simulink model "TDsimulation"  (Simulink 8.3)
settings: Solver=ode4  StartTime=0.0  StopTime=Tsim  FixedStep=Ts  RelTol=1e-3
InitFcn:
  | GlobalParam;
values from neighbouring files (symbols this model uses):
  APFon = 0.02    [GlobalParam.m]
  Cdc = 680e-6    (= 0.00068)    [GlobalParam.m]
  fe = 50    [GlobalParam.m]
  Ideal = 0    [GlobalParam.m]
  Lf = 0.002996    [GlobalParam.m]
  LL = 0.055462    [GlobalParam.m]
  Rf = 0.09    [GlobalParam.m]
  RL = 23.232    [GlobalParam.m]
  tetaa = 0    [GlobalParam.m]
  tetab = -120    [GlobalParam.m]
  tetac = 120    [GlobalParam.m]
  Tm = 1/fm    (= 0.0001)    [GlobalParam.m]
  Ts = 1e-6    (= 1e-06)    [GlobalParam.m]
  Vdc = 114    [GlobalParam.m]
  Vs = 310.2    [GlobalParam.m]
libraries: powerlib x115, powerlib_extras x3
(part 1 of 2)
settings Model: Creator=User  LastModifiedBy=Leocompa
settings OptimizationCC: ExpressionDepthLimit=2147483647
settings DebuggingCC: FcnCallInpInsideContextMsg=EnableAllAsWarning
settings GRTTargetCC: CombineOutputUpdateFcns=on  GRTInterface=off

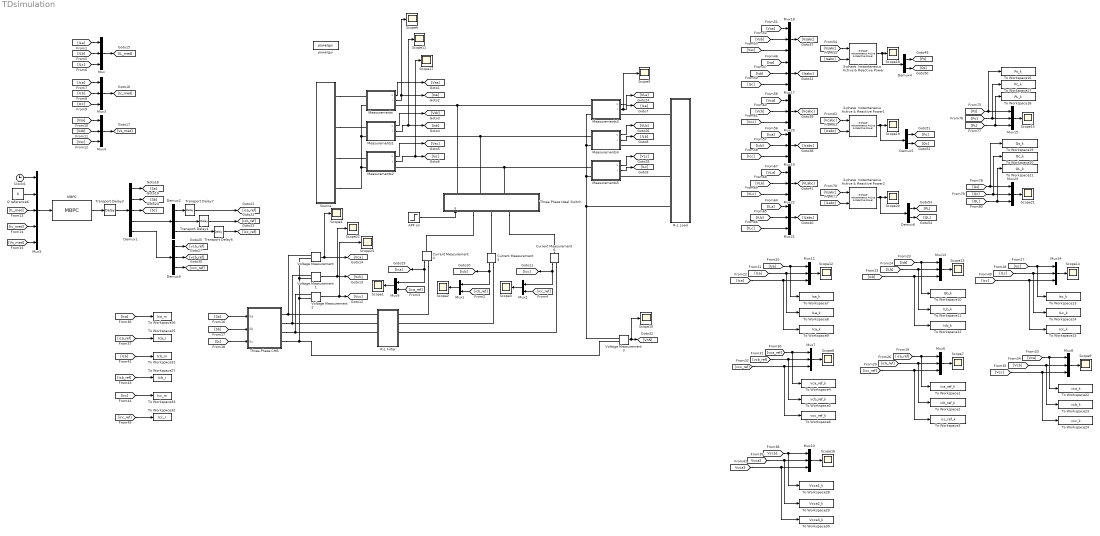
== system TDsimulation ==
  3-phase  Instantaneous  Active & Reactive Power : powerlib_extras/Measurements/3-phase  Instantaneous  Active & Reactive Power
  3-phase  Instantaneous  Active & Reactive Power1 : powerlib_extras/Measurements/3-phase  Instantaneous  Active & Reactive Power
  3-phase  Instantaneous  Active & Reactive Power2 : powerlib_extras/Measurements/3-phase  Instantaneous  Active & Reactive Power
  APF on : Step  Time=APFon  SampleTime=0
  Clock6 : Clock
  Current Measurement4 : powerlib/Measurements/Current Measurement  PhasorSimulation=off  OutputType=Complex  PSBequivalent=0
  Current Measurement5 : powerlib/Measurements/Current Measurement  PhasorSimulation=off  OutputType=Complex  PSBequivalent=0
  Current Measurement6 : powerlib/Measurements/Current Measurement  PhasorSimulation=off  OutputType=Complex  PSBequivalent=0
  Demux1 : Demux  Outputs=5
  Demux2 : Demux  Outputs=3
  Demux4 : Demux  Outputs=2
  Demux5 : Demux  Outputs=2
  Demux6 : Demux  Outputs=2
  Demux9 : Demux  Outputs=3
  MBPC : MATLABFcn  MATLABFcn=MBPC  OutputDimensions=24
  Measurements : Subsystem
  Measurements1 : Subsystem
  Measurements2 : Subsystem
  Measurements3 : Subsystem
  Measurements4 : Subsystem
  Measurements5 : Subsystem
  Mux{,3..4,6..8,10,12..15,17..23} (18 alike) : Mux  Inputs=3
  Mux1 : Mux  Inputs=2
  Mux2 : Mux  Inputs=2
  Mux5 : Mux  Inputs=5
  Mux9 : Mux  Inputs=2
  Q reference6 : Constant  Value=0
  R-L Filter : Subsystem
  R-L Load : Subsystem
  Scope{1..23} (23 alike) : Scope
      Scope1 settings: YMin=-15  YMax=65  SaveName=Vo
      Scope10 settings: YMin=-2500  YMax=37500  SaveName=vNn
      Scope11 settings: YMin=-10.7  YMax=-9.4  SaveName=isb
      Scope12 settings: YMin=-11  YMax=11  SaveName=Vo11
      Scope13 settings: YMin=-11  YMax=11  SaveName=Vo12
      Scope14 settings: YMin=25  YMax=575  SaveName=Vo13
      Scope15 settings: YMin=-750  YMax=4250  SaveName=Vo14
      Scope16 settings: TimeRange=0.1  YMin=27.5  YMax=75  SaveName=Vo15
      Scope17 settings: YMin=-10.7  YMax=-9.4  SaveName=isc
      Scope18 settings: YMin=-1500  YMax=5500  SaveName=Vo17
      Scope19 settings: YMin=-1500  YMax=5500  SaveName=Vo18
      Scope2 settings: YMin=-2.5  YMax=6.5  SaveName=Vo1
      Scope20 settings: YMin=-1500  YMax=5500  SaveName=Vo19
      Scope21 settings: TimeRange=0.1  YMin=-400  YMax=4000  SaveName=Vo20
      Scope22 settings: YMin=-2500  YMax=37500  SaveName=vcb
      Scope23 settings: YMin=-2500  YMax=37500  SaveName=vcc
      Scope3 settings: YMin=-2.5  YMax=6.5  SaveName=Vo2
      Scope4 settings: YMin=-2500  YMax=37500  SaveName=vca
      Scope5 settings: YMin=-2500  YMax=37500  SaveName=iLa
      Scope6 settings: YMin=-10.7  YMax=-9.4  SaveName=isa
      Scope7 settings: YMin=25  YMax=575  SaveName=Vo6
      Scope8 settings: YMin=25  YMax=575  SaveName=Vo7
      Scope9 settings: YMin=25  YMax=575  SaveName=Vo8
  Source : Subsystem
  Three-Phase CHB : Subsystem
  Three-Phase Ideal Switch : Subsystem
  To Workspace1 : ToWorkspace  VariableName=ica_ref_k  SaveFormat=Timeseries  SampleTime=-1
  To Workspace10 : ToWorkspace  VariableName=Isb_k  SaveFormat=Timeseries  SampleTime=-1
  To Workspace11 : ToWorkspace  VariableName=ILb_k  SaveFormat=Timeseries  SampleTime=-1
  To Workspace12 : ToWorkspace  VariableName=Icb_k  SaveFormat=Timeseries  SampleTime=-1
  To Workspace13 : ToWorkspace  VariableName=Isc_k  SaveFormat=Timeseries  SampleTime=-1
  To Workspace14 : ToWorkspace  VariableName=ILc_k  SaveFormat=Timeseries  SampleTime=-1
  To Workspace15 : ToWorkspace  VariableName=Icc_k  SaveFormat=Timeseries  SampleTime=-1
  To Workspace16 : ToWorkspace  VariableName=Ps_k  SaveFormat=Timeseries  SampleTime=-1
  To Workspace17 : ToWorkspace  VariableName=Pc_k  SaveFormat=Timeseries  SampleTime=-1
  To Workspace18 : ToWorkspace  VariableName=PL_k  SaveFormat=Timeseries  SampleTime=-1
  To Workspace19 : ToWorkspace  VariableName=Qs_k  SaveFormat=Timeseries  SampleTime=-1
  To Workspace2 : ToWorkspace  VariableName=icb_ref_k  SaveFormat=Timeseries  SampleTime=-1
  To Workspace20 : ToWorkspace  VariableName=Qc_k  SaveFormat=Timeseries  SampleTime=-1
  To Workspace21 : ToWorkspace  VariableName=QL_k  SaveFormat=Timeseries  SampleTime=-1
  To Workspace22 : ToWorkspace  VariableName=vca_k  SaveFormat=Timeseries  SampleTime=-1
  To Workspace23 : ToWorkspace  VariableName=vcb_k  SaveFormat=Timeseries  SampleTime=-1
  To Workspace24 : ToWorkspace  VariableName=vcc_k  SaveFormat=Timeseries  SampleTime=-1
  To Workspace25 : ToWorkspace  VariableName=Ica_r  SampleTime=-1
  To Workspace26 : ToWorkspace  VariableName=Ica_m  SampleTime=-1
  To Workspace27 : ToWorkspace  VariableName=Icb_r  SampleTime=-1
  To Workspace28 : ToWorkspace  VariableName=Vcca1_k  SaveFormat=Timeseries  SampleTime=-1
  To Workspace29 : ToWorkspace  VariableName=Vcca2_k  SaveFormat=Timeseries  SampleTime=-1
  To Workspace3 : ToWorkspace  VariableName=icc_ref_k  SaveFormat=Timeseries  SampleTime=-1
  To Workspace30 : ToWorkspace  VariableName=Vcca3_k  SaveFormat=Timeseries  SampleTime=-1
  To Workspace31 : ToWorkspace  VariableName=Icb_m  SampleTime=-1
  To Workspace32 : ToWorkspace  VariableName=Icc_r  SampleTime=-1
  To Workspace33 : ToWorkspace  VariableName=Icc_m  SampleTime=-1
  To Workspace4 : ToWorkspace  VariableName=vca_ref_k  SaveFormat=Timeseries  SampleTime=-1
  To Workspace5 : ToWorkspace  VariableName=vcb_ref_k  SaveFormat=Timeseries  SampleTime=-1
  To Workspace6 : ToWorkspace  VariableName=vcc_ref_k  SaveFormat=Timeseries  SampleTime=-1
  To Workspace7 : ToWorkspace  VariableName=Isa_k  SaveFormat=Timeseries  SampleTime=-1
  To Workspace8 : ToWorkspace  VariableName=ILa_k  SaveFormat=Timeseries  SampleTime=-1
  To Workspace9 : ToWorkspace  VariableName=Ica_k  SaveFormat=Timeseries  SampleTime=-1
  Transport Delay{3..4,6..7} (4 alike) : TransportDelay  DelayTime=Tm
  Voltage Measurement{,1..3} (4 alike) : powerlib/Measurements/Voltage Measurement  PhasorSimulation=off  OutputType=Complex  PSBequivalent=0
  powergui : powerlib/powergui  SimulationMode=Discrete  SolverType=Backward Euler  SampleTime=Ts  frequency=60  SPID=off  DisableSnubberDevices=off  DisableRonSwitches=off  DisableVfSwitches=off  SwTol=0  Interpol=off  DisplayEquations=off  Ts=0  methode=off  frequencyindice=0  Pbase=100e6  ErrMax=1e-4  Iterations=50  UnitsV=kV  UnitsW=MW  FunctionMessages=off  echomessages=off  HookPort=off  EnableUseOfTLC=off  x0status=blocks  RestoreLinks=warning  ResistiveCurrentMeasurement=off  Frange=[0:2:500]  Ylog=off  Xlog=on  ShowGrid=off  save=off  variable=ZData  structure=vcc  ZoomFFT=off  StartTime=0.03  cycles=2  DisplayStyle=1  fundamental=50  FreqAxis=off  MaxFrequency=60000  frequencyindicesteady=1  RmsSteady=1  display=off
  wires:
  Measurements/2(i) -> Scope6/1, [Isa]
  Measurements/1(v) -> [Vsa]
  Measurements1/1(v) -> [Vsb]
  Measurements2/1(v) -> [Vsc]
  Current Measurement4/1 -> Mux9/1, [Ica]
  Mux9/1 -> Scope1/1
  [ica_ref] -> Mux9/2
  Current Measurement5/1 -> Mux1/1, [Icb]
  Mux1/1 -> Scope2/1
  [icb_ref] -> Mux1/2
  Current Measurement6/1 -> Mux2/1, [Icc]
  Mux2/1 -> Scope3/1
  [icc_ref] -> Mux2/2
  Voltage Measurement/1 -> [Vca], Scope4/1
  Voltage Measurement2/1 -> Scope23/1, [Vcc]
  APF on/1 -> Three-Phase Ideal Switch/1(g)
  [ILa] -> Mux/1
  [ILb] -> Mux/2
  [ILc] -> Mux/3
  [Ica] -> Mux3/1
  [Icb] -> Mux3/2
  [Icc] -> Mux3/3
  [Vsa] -> Mux4/1
  [Vsb] -> Mux4/2
  [Vsc] -> Mux4/3
  Mux/1 -> [IL_med]
  Mux3/1 -> [Ic_med]
  Mux4/1 -> [Vs_med]
  [Sa] -> Three-Phase CHB/1(Sa)
  [Sb] -> Three-Phase CHB/2(Sb)
  [Sc] -> Three-Phase CHB/3(Sc)
  [Icb] -> Mux13/3, To Workspace12/1
  Mux12/1 -> Scope12/1
  Mux13/1 -> Scope13/1
  [Isc] -> Mux14/1, To Workspace13/1
  [Ica] -> Mux12/3, To Workspace9/1
  [ILc] -> Mux14/2, To Workspace14/1
  [Isa] -> Mux12/1, To Workspace7/1
  [ILb] -> Mux13/2, To Workspace11/1
  Mux14/1 -> Scope14/1
  [Icc] -> Mux14/3, To Workspace15/1
  [ILa] -> Mux12/2, To Workspace8/1
  [Isb] -> Mux13/1, To Workspace10/1
  [ica_ref] -> Mux6/1, To Workspace1/1
  [icb_ref] -> Mux6/2, To Workspace2/1
  Mux6/1 -> Scope7/1
  [icc_ref] -> Mux6/3, To Workspace3/1
  Demux6/1 -> [PL]
  Demux5/1 -> [Pc]
  Demux5/2 -> [Qc]
  [Isabc] -> 3-phase  Instantaneous  Active & Reactive Power/2
  [Vsb] -> Mux18/2
  [Ica] -> Mux19/1
  Mux17/1 -> [Isabc]
  Demux6/2 -> [QL]
  Demux4/1 -> [Ps]
  Demux4/2 -> [Qs]
  [ILc] -> Mux21/3
  Mux19/1 -> [Icabc]
  [PL] -> Mux15/3, To Workspace18/1
  [Pc] -> Mux15/2, To Workspace17/1
  [Icc] -> Mux19/3
  [Qc] -> Mux23/2, To Workspace20/1
  Mux21/1 -> [ILabc]
  [Qs] -> Mux23/1, To Workspace19/1
  [Isb] -> Mux17/2
  Mux18/1 -> [Vsabc]
  [Isc] -> Mux17/3
  [Vsabc] -> 3-phase  Instantaneous  Active & Reactive Power/1
  [ILa] -> Mux21/1
  Mux20/1 -> [Vcabc]
  [ILb] -> Mux21/2
  3-phase  Instantaneous  Active & Reactive Power2/1 -> Scope20/1, Demux6/1
  3-phase  Instantaneous  Active & Reactive Power1/1 -> Scope19/1, Demux5/1
  Mux22/1 -> [VLabc]
  [Vsa] -> Mux18/1
  [Vsabc] -> 3-phase  Instantaneous  Active & Reactive Power2/1
  Mux15/1 -> Scope15/1
  [ILabc] -> 3-phase  Instantaneous  Active & Reactive Power2/2
  [Vcc] -> Mux20/3
  Mux23/1 -> Scope21/1
  [Icabc] -> 3-phase  Instantaneous  Active & Reactive Power1/2
  [Icb] -> Mux19/2
  [VLc] -> Mux22/3
  [Isa] -> Mux17/1
  [Vcb] -> Mux20/2
  [Vsc] -> Mux18/3
  [Vca] -> Mux20/1
  [VLa] -> Mux22/1
  [Ps] -> Mux15/1, To Workspace16/1
  [VLb] -> Mux22/2
  3-phase  Instantaneous  Active & Reactive Power/1 -> Scope18/1, Demux4/1
  [QL] -> Mux23/3, To Workspace21/1
  [Vcabc] -> 3-phase  Instantaneous  Active & Reactive Power1/1
  Measurements3/2(i) -> Scope5/1, [ILa]
  Measurements3/1(v) -> [VLa]
  Measurements4/2(i) -> [ILb]
  Measurements4/1(v) -> [VLb]
  Measurements5/2(i) -> [ILc]
  Measurements5/1(v) -> [VLc]
  [vca_ref] -> Mux7/1, To Workspace4/1
  [vcb_ref] -> Mux7/2, To Workspace5/1
  Mux7/1 -> Scope8/1
  [vcc_ref] -> Mux7/3, To Workspace6/1
  [Vca] -> Mux8/1, To Workspace22/1
  [Vcb] -> Mux8/2, To Workspace23/1
  Mux8/1 -> Scope9/1
  [Vcc] -> Mux8/3, To Workspace24/1
  Voltage Measurement3/1 -> Scope10/1, [VnN]
  [Ica] -> To Workspace26/1
  [ica_ref] -> To Workspace25/1
  Mux10/1 -> Scope16/1
  [Vcca1] -> Mux10/1, To Workspace28/1
  [Vcca2] -> Mux10/2, To Workspace29/1
  [Vcca3] -> Mux10/3, To Workspace30/1
  Measurements1/2(i) -> Scope11/1, [Isb]
  Measurements2/2(i) -> [Isc], Scope17/1
  [Icb] -> To Workspace31/1
  [icb_ref] -> To Workspace27/1
  [Icc] -> To Workspace33/1
  [icc_ref] -> To Workspace32/1
  Voltage Measurement1/1 -> [Vcb], Scope22/1
  Mux5/1 -> MBPC/1
  [IL_med] -> Mux5/3
  [Ic_med] -> Mux5/4
  [Vs_med] -> Mux5/5
  Q reference6/1 -> Mux5/2
  Clock6/1 -> Mux5/1
  Demux9/3 -> [vcc_ref]
  Demux9/2 -> [vcb_ref]
  Demux9/1 -> [vca_ref]
  Demux1/1 -> [Sa]
  Demux1/2 -> [Sb]
  Demux1/3 -> [Sc]
  Demux1/4 -> Demux2/1
  Demux1/5 -> Demux9/1
  Transport Delay3/1 -> Demux1/1
  MBPC/1 -> Transport Delay3/1
  Demux2/1 -> Transport Delay7/1
  Demux2/2 -> Transport Delay4/1
  Demux2/3 -> Transport Delay6/1
  Transport Delay6/1 -> [icc_ref]
  Transport Delay7/1 -> [ica_ref]
  Transport Delay4/1 -> [icb_ref]
  connections:
  Source/RConn3 -- Measurements2/LConn1
  Source/RConn2 -- Measurements1/LConn1
  Source/RConn1 -- Measurements/LConn1
  Measurements/LConn2 -- Source/RConn4 -- Measurements2/LConn2 -- Measurements1/LConn2
  Three-Phase Ideal Switch/RConn1 -- Measurements3/LConn1 -- Measurements/RConn1
  Three-Phase Ideal Switch/RConn2 -- Measurements4/LConn1 -- Measurements1/RConn1
  Three-Phase Ideal Switch/RConn3 -- Measurements5/LConn1 -- Measurements2/RConn1
  Current Measurement4/RConn1 -- R-L Filter/RConn1
  Current Measurement5/RConn1 -- R-L Filter/RConn2
  Current Measurement6/RConn1 -- R-L Filter/RConn3
  Three-Phase Ideal Switch/LConn2 -- Current Measurement5/LConn1
  Three-Phase Ideal Switch/LConn3 -- Current Measurement6/LConn1
  Three-Phase Ideal Switch/LConn1 -- Current Measurement4/LConn1
  Voltage Measurement/LConn2 -- Voltage Measurement1/LConn2 -- Voltage Measurement2/LConn2 -- Voltage Measurement3/LConn2 -- Three-Phase CHB/RConn4
  Three-Phase CHB/RConn3 -- R-L Filter/LConn3 -- Voltage Measurement2/LConn1
  Three-Phase CHB/RConn2 -- R-L Filter/LConn2 -- Voltage Measurement1/LConn1
  Three-Phase CHB/RConn1 -- R-L Filter/LConn1 -- Voltage Measurement/LConn1
  Measurements4/LConn2 -- R-L Load/LConn4 -- Voltage Measurement3/LConn1 -- Measurements5/LConn2 -- Measurements3/LConn2
  R-L Load/LConn3 -- Measurements5/RConn1
  R-L Load/LConn2 -- Measurements4/RConn1
  R-L Load/LConn1 -- Measurements3/RConn1

== system TDsimulation/Measurements ==
  Current Measurement : powerlib/Measurements/Current Measurement  PhasorSimulation=off  OutputType=Complex  PSBequivalent=0
  Voltage Measurement : powerlib/Measurements/Voltage Measurement  PhasorSimulation=off  OutputType=Complex  PSBequivalent=0
  vi+ : PMIOPort  Port=1  Side=Left
  i- : PMIOPort  Port=2  Side=Right
  v- : PMIOPort  Port=3  Side=Left
  v : Outport
  i : Outport  Port=2
  wires:
  Current Measurement/1 -> i/1
  Voltage Measurement/1 -> v/1
  connections:
  Voltage Measurement/LConn1 -- Current Measurement/LConn1 -- vi+/RConn1
  Current Measurement/RConn1 -- i-/RConn1
  Voltage Measurement/LConn2 -- v-/RConn1

== system TDsimulation/Measurements1 ==
  Current Measurement : powerlib/Measurements/Current Measurement  PhasorSimulation=off  OutputType=Complex  PSBequivalent=0
  Voltage Measurement : powerlib/Measurements/Voltage Measurement  PhasorSimulation=off  OutputType=Complex  PSBequivalent=0
  vi+ : PMIOPort  Port=1  Side=Left
  i- : PMIOPort  Port=2  Side=Right
  v- : PMIOPort  Port=3  Side=Left
  v : Outport
  i : Outport  Port=2
  wires:
  Current Measurement/1 -> i/1
  Voltage Measurement/1 -> v/1
  connections:
  Voltage Measurement/LConn1 -- vi+/RConn1 -- Current Measurement/LConn1
  Current Measurement/RConn1 -- i-/RConn1
  Voltage Measurement/LConn2 -- v-/RConn1

== system TDsimulation/Measurements2 ==
  Current Measurement : powerlib/Measurements/Current Measurement  PhasorSimulation=off  OutputType=Complex  PSBequivalent=0
  Voltage Measurement : powerlib/Measurements/Voltage Measurement  PhasorSimulation=off  OutputType=Complex  PSBequivalent=0
  vi+ : PMIOPort  Port=1  Side=Left
  i- : PMIOPort  Port=2  Side=Right
  v- : PMIOPort  Port=3  Side=Left
  v : Outport
  i : Outport  Port=2
  wires:
  Current Measurement/1 -> i/1
  Voltage Measurement/1 -> v/1
  connections:
  Voltage Measurement/LConn1 -- vi+/RConn1 -- Current Measurement/LConn1
  Current Measurement/RConn1 -- i-/RConn1
  Voltage Measurement/LConn2 -- v-/RConn1

== system TDsimulation/Measurements3 ==
  Current Measurement : powerlib/Measurements/Current Measurement  PhasorSimulation=off  OutputType=Complex  PSBequivalent=0
  Voltage Measurement : powerlib/Measurements/Voltage Measurement  PhasorSimulation=off  OutputType=Complex  PSBequivalent=0
  vi+ : PMIOPort  Port=1  Side=Left
  i- : PMIOPort  Port=2  Side=Right
  v- : PMIOPort  Port=3  Side=Left
  v : Outport
  i : Outport  Port=2
  wires:
  Current Measurement/1 -> i/1
  Voltage Measurement/1 -> v/1
  connections:
  Voltage Measurement/LConn1 -- vi+/RConn1 -- Current Measurement/LConn1
  Current Measurement/RConn1 -- i-/RConn1
  Voltage Measurement/LConn2 -- v-/RConn1

== system TDsimulation/Measurements4 ==
  Current Measurement : powerlib/Measurements/Current Measurement  PhasorSimulation=off  OutputType=Complex  PSBequivalent=0
  Voltage Measurement : powerlib/Measurements/Voltage Measurement  PhasorSimulation=off  OutputType=Complex  PSBequivalent=0
  vi+ : PMIOPort  Port=1  Side=Left
  i- : PMIOPort  Port=2  Side=Right
  v- : PMIOPort  Port=3  Side=Left
  v : Outport
  i : Outport  Port=2
  wires:
  Current Measurement/1 -> i/1
  Voltage Measurement/1 -> v/1
  connections:
  Voltage Measurement/LConn1 -- vi+/RConn1 -- Current Measurement/LConn1
  Current Measurement/RConn1 -- i-/RConn1
  Voltage Measurement/LConn2 -- v-/RConn1

== system TDsimulation/Measurements5 ==
  Current Measurement : powerlib/Measurements/Current Measurement  PhasorSimulation=off  OutputType=Complex  PSBequivalent=0
  Voltage Measurement : powerlib/Measurements/Voltage Measurement  PhasorSimulation=off  OutputType=Complex  PSBequivalent=0
  vi+ : PMIOPort  Port=1  Side=Left
  i- : PMIOPort  Port=2  Side=Right
  v- : PMIOPort  Port=3  Side=Left
  v : Outport
  i : Outport  Port=2
  wires:
  Current Measurement/1 -> i/1
  Voltage Measurement/1 -> v/1
  connections:
  Voltage Measurement/LConn1 -- vi+/RConn1 -- Current Measurement/LConn1
  Current Measurement/RConn1 -- i-/RConn1
  Voltage Measurement/LConn2 -- v-/RConn1

== system TDsimulation/R-L Filter ==
  RL{1..4} (4 alike) : powerlib/Elements/Series RLC Branch  LConnTagsString=__new0  RConnTagsString=__new0  BranchType=RL  Resistance=Rf  Inductance=Lf  SetiL0=off  InitialCurrent=0  Capacitance=1e-6  Setx0=off  InitialVoltage=0  Measurements=None
  ai : PMIOPort  Port=1  Side=Left
  bi : PMIOPort  Port=2  Side=Left
  ci : PMIOPort  Port=3  Side=Left
  ao : PMIOPort  Port=4  Side=Right
  bo : PMIOPort  Port=5  Side=Right
  co : PMIOPort  Port=6  Side=Right
  ni : PMIOPort  Port=7  Side=Left
  no : PMIOPort  Port=8  Side=Right
  connections:
  RL3/LConn1 -- ci/RConn1
  RL2/LConn1 -- bi/RConn1
  RL1/LConn1 -- ai/RConn1
  ao/RConn1 -- RL1/RConn1
  bo/RConn1 -- RL2/RConn1
  co/RConn1 -- RL3/RConn1
  no/RConn1 -- RL4/RConn1
  RL4/LConn1 -- ni/RConn1

== system TDsimulation/R-L Load ==
  RL1 : powerlib/Elements/Series RLC Branch  LConnTagsString=__new0  RConnTagsString=__new0  BranchType=RL  Resistance=RL  Inductance=LL  SetiL0=off  InitialCurrent=0  Capacitance=1e-6  Setx0=off  InitialVoltage=0  Measurements=None
  RL2 : powerlib/Elements/Series RLC Branch  LConnTagsString=__new0  RConnTagsString=__new0  BranchType=RL  Resistance=RL  Inductance=LL  SetiL0=off  InitialCurrent=0  Capacitance=1e-6  Setx0=off  InitialVoltage=0  Measurements=None
  RL3 : powerlib/Elements/Series RLC Branch  LConnTagsString=__new0  RConnTagsString=__new0  BranchType=RL  Resistance=RL  Inductance=LL  SetiL0=off  InitialCurrent=0  Capacitance=1e-6  Setx0=off  InitialVoltage=0  Measurements=None
  a : PMIOPort  Port=1  Side=Left
  b : PMIOPort  Port=2  Side=Left
  c : PMIOPort  Port=3  Side=Left
  n : PMIOPort  Port=4  Side=Left
  connections:
  RL2/RConn1 -- RL1/RConn1 -- n/RConn1 -- RL3/RConn1
  RL3/LConn1 -- c/RConn1
  RL2/LConn1 -- b/RConn1
  RL1/LConn1 -- a/RConn1

== system TDsimulation/Source ==
  Vsa : powerlib/Electrical Sources/AC Voltage Source  Amplitude=Vs  Phase=tetaa  Frequency=fe  SampleTime=0  Measurements=None
  Vsb : powerlib/Electrical Sources/AC Voltage Source  Amplitude=Vs  Phase=tetab  Frequency=fe  SampleTime=0  Measurements=None
  Vsc : powerlib/Electrical Sources/AC Voltage Source  Amplitude=Vs  Phase=tetac  Frequency=fe  SampleTime=0  Measurements=None
  a : PMIOPort  Port=1  Side=Right
  b : PMIOPort  Port=2  Side=Right
  c : PMIOPort  Port=3  Side=Right
  n : PMIOPort  Port=4  Side=Right
  connections:
  Vsc/RConn1 -- c/RConn1
  Vsa/LConn1 -- n/RConn1 -- Vsc/LConn1 -- Vsb/LConn1
  Vsb/RConn1 -- b/RConn1
  Vsa/RConn1 -- a/RConn1

== system TDsimulation/Three-Phase CHB ==
  Sa : Inport
  Sb : Inport  Port=2
  Sc : Inport  Port=3
  Demux : Demux  Outputs=6
  Demux1 : Demux  Outputs=6
  Demux2 : Demux  Outputs=6
  Single-Phase CHB1 : Subsystem
  Single-Phase CHB2 : Subsystem
  Single-Phase CHB3 : Subsystem
  a : PMIOPort  Port=1  Side=Right
  b : PMIOPort  Port=2  Side=Right
  c : PMIOPort  Port=3  Side=Right
  n : PMIOPort  Port=4  Side=Right
  wires:
  Demux/4 -> Single-Phase CHB1/4(sf23)
  Demux/6 -> Single-Phase CHB1/6(sf33)
  Demux/3 -> Single-Phase CHB1/3(sf21)
  Demux/2 -> Single-Phase CHB1/2(sf13)
  Demux/1 -> Single-Phase CHB1/1(sf11)
  Demux1/3 -> Single-Phase CHB2/3(sf21)
  Sa/1 -> Demux/1
  Sb/1 -> Demux1/1
  Sc/1 -> Demux2/1
  Demux2/1 -> Single-Phase CHB3/1(sf11)
  Demux1/1 -> Single-Phase CHB2/1(sf11)
  Demux1/6 -> Single-Phase CHB2/6(sf33)
  Demux2/6 -> Single-Phase CHB3/6(sf33)
  Demux/5 -> Single-Phase CHB1/5(sf31)
  Demux1/2 -> Single-Phase CHB2/2(sf13)
  Demux2/5 -> Single-Phase CHB3/5(sf31)
  Demux1/4 -> Single-Phase CHB2/4(sf23)
  Demux2/4 -> Single-Phase CHB3/4(sf23)
  Demux1/5 -> Single-Phase CHB2/5(sf31)
  Demux2/3 -> Single-Phase CHB3/3(sf21)
  Demux2/2 -> Single-Phase CHB3/2(sf13)
  connections:
  Single-Phase CHB2/RConn1 -- b/RConn1
  Single-Phase CHB1/RConn2 -- n/RConn1 -- Single-Phase CHB3/RConn2 -- Single-Phase CHB2/RConn2
  Single-Phase CHB1/RConn1 -- a/RConn1
  Single-Phase CHB3/RConn1 -- c/RConn1

== system TDsimulation/Three-Phase Ideal Switch ==
  g : Inport
  Ideal Switch{,1..3} (4 alike) : powerlib/Power Electronics/Ideal Switch  Ron=0.001  Lon=0  IC=0  Rs=1e5  Cs=inf  Measurements=on
  ao : PMIOPort  Port=1  Side=Right
  bo : PMIOPort  Port=2  Side=Right
  co : PMIOPort  Port=3  Side=Right
  ai : PMIOPort  Port=4  Side=Left
  bi : PMIOPort  Port=5  Side=Left
  ci : PMIOPort  Port=6  Side=Left
  no : PMIOPort  Port=7  Side=Left
  ni : PMIOPort  Port=8  Side=Right
  wires:
  g/1 -> Ideal Switch3/1, Ideal Switch2/1, Ideal Switch1/1, Ideal Switch/1
  connections:
  Ideal Switch1/RConn1 -- bo/RConn1
  Ideal Switch1/LConn1 -- bi/RConn1
  Ideal Switch/RConn1 -- ao/RConn1
  Ideal Switch2/RConn1 -- co/RConn1
  Ideal Switch2/LConn1 -- ci/RConn1
  Ideal Switch/LConn1 -- ai/RConn1
  Ideal Switch3/LConn1 -- ni/RConn1
  Ideal Switch3/RConn1 -- no/RConn1

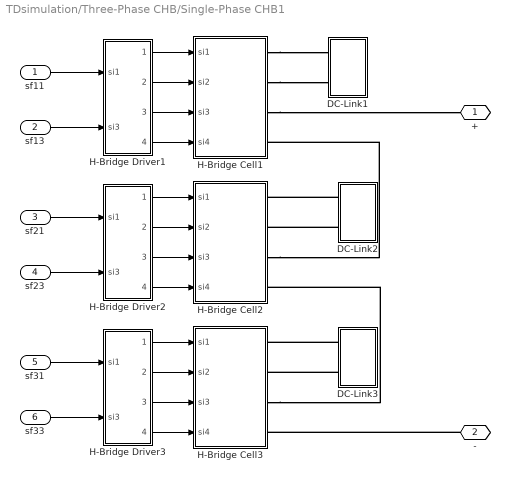
== system TDsimulation/Three-Phase CHB/Single-Phase CHB1 ==
  sf11 : Inport
  sf13 : Inport  Port=2
  sf21 : Inport  Port=3
  sf23 : Inport  Port=4
  sf31 : Inport  Port=5
  sf33 : Inport  Port=6
  DC-Link1 : Subsystem
  DC-Link2 : Subsystem
  DC-Link3 : Subsystem
  H-Bridge Cell1 : Subsystem
  H-Bridge Cell2 : Subsystem
  H-Bridge Cell3 : Subsystem
  H-Bridge Driver1 : Subsystem
  H-Bridge Driver2 : Subsystem
  H-Bridge Driver3 : Subsystem
  + : PMIOPort  Port=1  Side=Right
  - : PMIOPort  Port=2  Side=Right
  wires:
  H-Bridge Driver2/1(1) -> H-Bridge Cell2/1(si1)
  H-Bridge Driver2/3(3) -> H-Bridge Cell2/3(si3)
  H-Bridge Driver2/2(2) -> H-Bridge Cell2/2(si2)
  H-Bridge Driver2/4(4) -> H-Bridge Cell2/4(si4)
  H-Bridge Driver1/1(1) -> H-Bridge Cell1/1(si1)
  H-Bridge Driver1/2(2) -> H-Bridge Cell1/2(si2)
  H-Bridge Driver1/3(3) -> H-Bridge Cell1/3(si3)
  H-Bridge Driver1/4(4) -> H-Bridge Cell1/4(si4)
  sf23/1 -> H-Bridge Driver2/2(si3)
  sf13/1 -> H-Bridge Driver1/2(si3)
  sf21/1 -> H-Bridge Driver2/1(si1)
  sf31/1 -> H-Bridge Driver3/1(si1)
  sf11/1 -> H-Bridge Driver1/1(si1)
  sf33/1 -> H-Bridge Driver3/2(si3)
  H-Bridge Driver3/2(2) -> H-Bridge Cell3/2(si2)
  H-Bridge Driver3/1(1) -> H-Bridge Cell3/1(si1)
  H-Bridge Driver3/3(3) -> H-Bridge Cell3/3(si3)
  H-Bridge Driver3/4(4) -> H-Bridge Cell3/4(si4)
  connections:
  H-Bridge Cell2/RConn3 -- H-Bridge Cell1/RConn4
  DC-Link2/RConn2 -- H-Bridge Cell2/RConn2
  DC-Link2/RConn1 -- H-Bridge Cell2/RConn1
  H-Bridge Cell1/RConn1 -- DC-Link1/RConn1
  H-Bridge Cell1/RConn2 -- DC-Link1/RConn2
  H-Bridge Cell1/RConn3 -- +/RConn1
  -/RConn1 -- H-Bridge Cell3/RConn4
  H-Bridge Cell3/RConn3 -- H-Bridge Cell2/RConn4
  DC-Link3/RConn2 -- H-Bridge Cell3/RConn2
  DC-Link3/RConn1 -- H-Bridge Cell3/RConn1

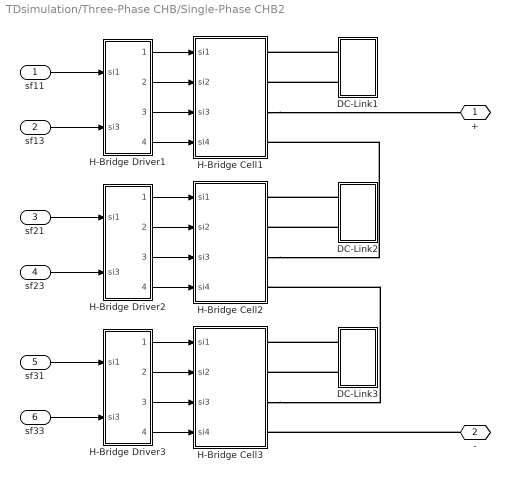
== system TDsimulation/Three-Phase CHB/Single-Phase CHB2 ==
  sf11 : Inport
  sf13 : Inport  Port=2
  sf21 : Inport  Port=3
  sf23 : Inport  Port=4
  sf31 : Inport  Port=5
  sf33 : Inport  Port=6
  DC-Link1 : Subsystem
  DC-Link2 : Subsystem
  DC-Link3 : Subsystem
  H-Bridge Cell1 : Subsystem
  H-Bridge Cell2 : Subsystem
  H-Bridge Cell3 : Subsystem
  H-Bridge Driver1 : Subsystem
  H-Bridge Driver2 : Subsystem
  H-Bridge Driver3 : Subsystem
  + : PMIOPort  Port=1  Side=Right
  - : PMIOPort  Port=2  Side=Right
  wires:
  H-Bridge Driver2/1(1) -> H-Bridge Cell2/1(si1)
  H-Bridge Driver2/3(3) -> H-Bridge Cell2/3(si3)
  H-Bridge Driver2/2(2) -> H-Bridge Cell2/2(si2)
  H-Bridge Driver2/4(4) -> H-Bridge Cell2/4(si4)
  H-Bridge Driver1/1(1) -> H-Bridge Cell1/1(si1)
  H-Bridge Driver1/2(2) -> H-Bridge Cell1/2(si2)
  H-Bridge Driver1/3(3) -> H-Bridge Cell1/3(si3)
  H-Bridge Driver1/4(4) -> H-Bridge Cell1/4(si4)
  sf23/1 -> H-Bridge Driver2/2(si3)
  sf13/1 -> H-Bridge Driver1/2(si3)
  sf21/1 -> H-Bridge Driver2/1(si1)
  sf31/1 -> H-Bridge Driver3/1(si1)
  sf11/1 -> H-Bridge Driver1/1(si1)
  sf33/1 -> H-Bridge Driver3/2(si3)
  H-Bridge Driver3/2(2) -> H-Bridge Cell3/2(si2)
  H-Bridge Driver3/1(1) -> H-Bridge Cell3/1(si1)
  H-Bridge Driver3/3(3) -> H-Bridge Cell3/3(si3)
  H-Bridge Driver3/4(4) -> H-Bridge Cell3/4(si4)
  connections:
  H-Bridge Cell2/RConn3 -- H-Bridge Cell1/RConn4
  DC-Link2/RConn2 -- H-Bridge Cell2/RConn2
  DC-Link2/RConn1 -- H-Bridge Cell2/RConn1
  DC-Link1/RConn1 -- H-Bridge Cell1/RConn1
  DC-Link1/RConn2 -- H-Bridge Cell1/RConn2
  H-Bridge Cell1/RConn3 -- +/RConn1
  -/RConn1 -- H-Bridge Cell3/RConn4
  H-Bridge Cell3/RConn3 -- H-Bridge Cell2/RConn4
  DC-Link3/RConn2 -- H-Bridge Cell3/RConn2
  DC-Link3/RConn1 -- H-Bridge Cell3/RConn1

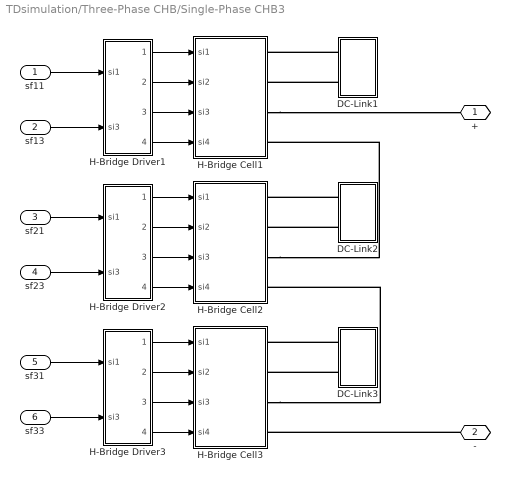
== system TDsimulation/Three-Phase CHB/Single-Phase CHB3 ==
  sf11 : Inport
  sf13 : Inport  Port=2
  sf21 : Inport  Port=3
  sf23 : Inport  Port=4
  sf31 : Inport  Port=5
  sf33 : Inport  Port=6
  DC-Link1 : Subsystem
  DC-Link2 : Subsystem
  DC-Link3 : Subsystem
  H-Bridge Cell1 : Subsystem
  H-Bridge Cell2 : Subsystem
  H-Bridge Cell3 : Subsystem
  H-Bridge Driver1 : Subsystem
  H-Bridge Driver2 : Subsystem
  H-Bridge Driver3 : Subsystem
  + : PMIOPort  Port=1  Side=Right
  - : PMIOPort  Port=2  Side=Right
  wires:
  H-Bridge Driver2/1(1) -> H-Bridge Cell2/1(si1)
  H-Bridge Driver2/3(3) -> H-Bridge Cell2/3(si3)
  H-Bridge Driver2/2(2) -> H-Bridge Cell2/2(si2)
  H-Bridge Driver2/4(4) -> H-Bridge Cell2/4(si4)
  H-Bridge Driver1/1(1) -> H-Bridge Cell1/1(si1)
  H-Bridge Driver1/2(2) -> H-Bridge Cell1/2(si2)
  H-Bridge Driver1/3(3) -> H-Bridge Cell1/3(si3)
  H-Bridge Driver1/4(4) -> H-Bridge Cell1/4(si4)
  sf23/1 -> H-Bridge Driver2/2(si3)
  sf13/1 -> H-Bridge Driver1/2(si3)
  sf21/1 -> H-Bridge Driver2/1(si1)
  sf31/1 -> H-Bridge Driver3/1(si1)
  sf11/1 -> H-Bridge Driver1/1(si1)
  sf33/1 -> H-Bridge Driver3/2(si3)
  H-Bridge Driver3/2(2) -> H-Bridge Cell3/2(si2)
  H-Bridge Driver3/1(1) -> H-Bridge Cell3/1(si1)
  H-Bridge Driver3/3(3) -> H-Bridge Cell3/3(si3)
  H-Bridge Driver3/4(4) -> H-Bridge Cell3/4(si4)
  connections:
  H-Bridge Cell2/RConn3 -- H-Bridge Cell1/RConn4
  DC-Link2/RConn2 -- H-Bridge Cell2/RConn2
  DC-Link2/RConn1 -- H-Bridge Cell2/RConn1
  DC-Link1/RConn1 -- H-Bridge Cell1/RConn1
  DC-Link1/RConn2 -- H-Bridge Cell1/RConn2
  H-Bridge Cell1/RConn3 -- +/RConn1
  -/RConn1 -- H-Bridge Cell3/RConn4
  H-Bridge Cell3/RConn3 -- H-Bridge Cell2/RConn4
  DC-Link3/RConn2 -- H-Bridge Cell3/RConn2
  DC-Link3/RConn1 -- H-Bridge Cell3/RConn1

== system TDsimulation/Three-Phase CHB/Single-Phase CHB1/DC-Link1 ==
  Constant : Constant  Value=Ideal
  DC Capacitor : powerlib/Elements/Series RLC Branch  LConnTagsString=__new0  RConnTagsString=__new0  BranchType=C  Resistance=0.09  Inductance=0.002996  SetiL0=off  InitialCurrent=0  Capacitance=Cdc  Setx0=on  InitialVoltage=Vodc  Measurements=None
  DC Voltage Source : powerlib/Electrical Sources/DC Voltage Source  Amplitude=Vdc  Measurements=None
  Ideal Switch : powerlib/Power Electronics/Ideal Switch  Ron=0.001  Lon=0  IC=0  Rs=1e5  Cs=inf  Measurements=on
  Ideal Switch1 : powerlib/Power Electronics/Ideal Switch  Ron=0.001  Lon=0  IC=0  Rs=1e5  Cs=inf  Measurements=on
  Logical Operator2 : Logic  Operator=NOT  AllPortsSameDT=off  OutDataTypeStr=boolean
  Vcan3 : powerlib/Measurements/Voltage Measurement  PhasorSimulation=off  OutputType=Complex  PSBequivalent=0
  + : PMIOPort  Port=1  Side=Right
  - : PMIOPort  Port=2  Side=Right
  tag scope: Vcca1=global
  wires:
  Constant/1 -> Ideal Switch/1, Logical Operator2/1
  Logical Operator2/1 -> Ideal Switch1/1
  Vcan3/1 -> [Vcca1]
  connections:
  DC Capacitor/LConn1 -- Ideal Switch1/LConn1
  Ideal Switch1/RConn1 -- Ideal Switch/RConn1 -- Vcan3/LConn1 -- +/RConn1
  DC Voltage Source/RConn1 -- Ideal Switch/LConn1
  -/RConn1 -- Vcan3/LConn2 -- DC Voltage Source/LConn1 -- DC Capacitor/RConn1

== system TDsimulation/Three-Phase CHB/Single-Phase CHB1/DC-Link2 ==
  Constant : Constant  Value=Ideal
  DC Capacitor : powerlib/Elements/Series RLC Branch  LConnTagsString=__new0  RConnTagsString=__new0  BranchType=C  Resistance=0.09  Inductance=0.002996  SetiL0=off  InitialCurrent=0  Capacitance=Cdc  Setx0=on  InitialVoltage=Vodc  Measurements=None
  DC Voltage Source : powerlib/Electrical Sources/DC Voltage Source  Amplitude=Vdc  Measurements=None
  Ideal Switch : powerlib/Power Electronics/Ideal Switch  Ron=0.001  Lon=0  IC=0  Rs=1e5  Cs=inf  Measurements=on
  Ideal Switch1 : powerlib/Power Electronics/Ideal Switch  Ron=0.001  Lon=0  IC=0  Rs=1e5  Cs=inf  Measurements=on
  Logical Operator2 : Logic  Operator=NOT  AllPortsSameDT=off  OutDataTypeStr=boolean
  Vcan3 : powerlib/Measurements/Voltage Measurement  PhasorSimulation=off  OutputType=Complex  PSBequivalent=0
  + : PMIOPort  Port=1  Side=Right
  - : PMIOPort  Port=2  Side=Right
  tag scope: Vcca2=global
  wires:
  Constant/1 -> Ideal Switch/1, Logical Operator2/1
  Logical Operator2/1 -> Ideal Switch1/1
  Vcan3/1 -> [Vcca2]
  connections:
  DC Capacitor/LConn1 -- Ideal Switch1/LConn1
  Ideal Switch1/RConn1 -- Ideal Switch/RConn1 -- Vcan3/LConn1 -- +/RConn1
  DC Voltage Source/RConn1 -- Ideal Switch/LConn1
  -/RConn1 -- DC Capacitor/RConn1 -- DC Voltage Source/LConn1 -- Vcan3/LConn2

== system TDsimulation/Three-Phase CHB/Single-Phase CHB1/DC-Link3 ==
  Constant : Constant  Value=Ideal
  DC Capacitor : powerlib/Elements/Series RLC Branch  LConnTagsString=__new0  RConnTagsString=__new0  BranchType=C  Resistance=0.09  Inductance=0.002996  SetiL0=off  InitialCurrent=0  Capacitance=Cdc  Setx0=on  InitialVoltage=Vodc  Measurements=None
  DC Voltage Source : powerlib/Electrical Sources/DC Voltage Source  Amplitude=Vdc  Measurements=None
  Ideal Switch : powerlib/Power Electronics/Ideal Switch  Ron=0.001  Lon=0  IC=0  Rs=1e5  Cs=inf  Measurements=on
  Ideal Switch1 : powerlib/Power Electronics/Ideal Switch  Ron=0.001  Lon=0  IC=0  Rs=1e5  Cs=inf  Measurements=on
  Logical Operator2 : Logic  Operator=NOT  AllPortsSameDT=off  OutDataTypeStr=boolean
  Vcan3 : powerlib/Measurements/Voltage Measurement  PhasorSimulation=off  OutputType=Complex  PSBequivalent=0
  + : PMIOPort  Port=1  Side=Right
  - : PMIOPort  Port=2  Side=Right
  tag scope: Vcca3=global
  wires:
  Constant/1 -> Ideal Switch/1, Logical Operator2/1
  Logical Operator2/1 -> Ideal Switch1/1
  Vcan3/1 -> [Vcca3]
  connections:
  DC Capacitor/LConn1 -- Ideal Switch1/LConn1
  Ideal Switch1/RConn1 -- Ideal Switch/RConn1 -- Vcan3/LConn1 -- +/RConn1
  DC Voltage Source/RConn1 -- Ideal Switch/LConn1
  -/RConn1 -- Vcan3/LConn2 -- DC Capacitor/RConn1 -- DC Voltage Source/LConn1

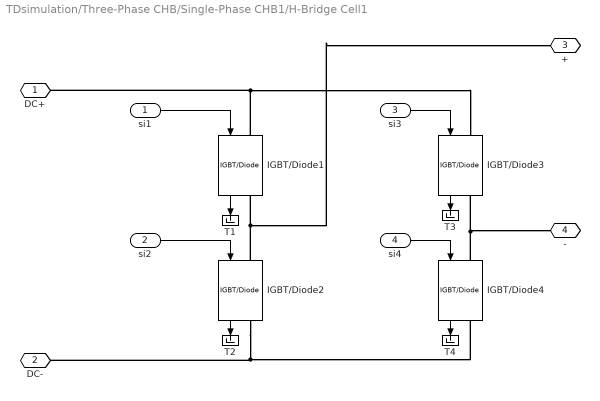
== system TDsimulation/Three-Phase CHB/Single-Phase CHB1/H-Bridge Cell1 ==
  si1 : Inport
  si2 : Inport  Port=2
  si3 : Inport  Port=3
  si4 : Inport  Port=4
  IGBT/Diode{1..4} (4 alike) : powerlib/Power Electronics/IGBT//Diode  Ron=1e-3  Rs=1e5  Cs=0.5  Measurements=on
  T{1..4} (4 alike) : Terminator
  DC+ : PMIOPort  Port=1  Side=Right
  DC- : PMIOPort  Port=2  Side=Right
  + : PMIOPort  Port=3  Side=Right
  - : PMIOPort  Port=4  Side=Right
  wires:
  si4/1 -> IGBT/Diode4/1
  si2/1 -> IGBT/Diode2/1
  si3/1 -> IGBT/Diode3/1
  si1/1 -> IGBT/Diode1/1
  IGBT/Diode1/1 -> T1/1
  IGBT/Diode2/1 -> T2/1
  IGBT/Diode4/1 -> T4/1
  IGBT/Diode3/1 -> T3/1
  connections:
  IGBT/Diode3/RConn1 -- IGBT/Diode4/LConn1 -- -/RConn1
  IGBT/Diode2/RConn1 -- IGBT/Diode4/RConn1 -- DC-/RConn1
  IGBT/Diode1/RConn1 -- IGBT/Diode2/LConn1 -- +/RConn1
  IGBT/Diode1/LConn1 -- IGBT/Diode3/LConn1 -- DC+/RConn1

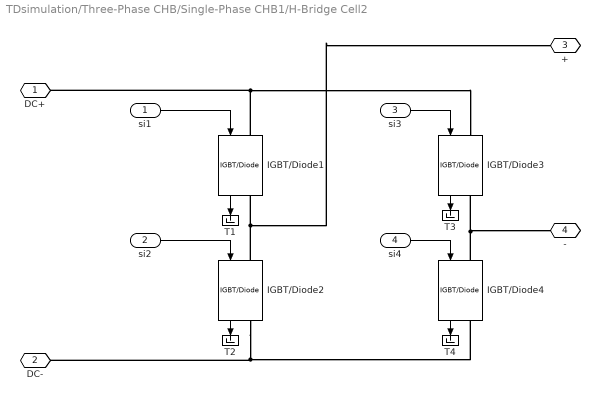
== system TDsimulation/Three-Phase CHB/Single-Phase CHB1/H-Bridge Cell2 ==
  si1 : Inport
  si2 : Inport  Port=2
  si3 : Inport  Port=3
  si4 : Inport  Port=4
  IGBT/Diode{1..4} (4 alike) : powerlib/Power Electronics/IGBT//Diode  Ron=1e-3  Rs=1e5  Cs=0.5  Measurements=on
  T{1..4} (4 alike) : Terminator
  DC+ : PMIOPort  Port=1  Side=Right
  DC- : PMIOPort  Port=2  Side=Right
  + : PMIOPort  Port=3  Side=Right
  - : PMIOPort  Port=4  Side=Right
  wires:
  si4/1 -> IGBT/Diode4/1
  si2/1 -> IGBT/Diode2/1
  si3/1 -> IGBT/Diode3/1
  si1/1 -> IGBT/Diode1/1
  IGBT/Diode1/1 -> T1/1
  IGBT/Diode2/1 -> T2/1
  IGBT/Diode4/1 -> T4/1
  IGBT/Diode3/1 -> T3/1
  connections:
  IGBT/Diode3/RConn1 -- IGBT/Diode4/LConn1 -- -/RConn1
  IGBT/Diode2/RConn1 -- IGBT/Diode4/RConn1 -- DC-/RConn1
  IGBT/Diode1/RConn1 -- IGBT/Diode2/LConn1 -- +/RConn1
  IGBT/Diode1/LConn1 -- IGBT/Diode3/LConn1 -- DC+/RConn1

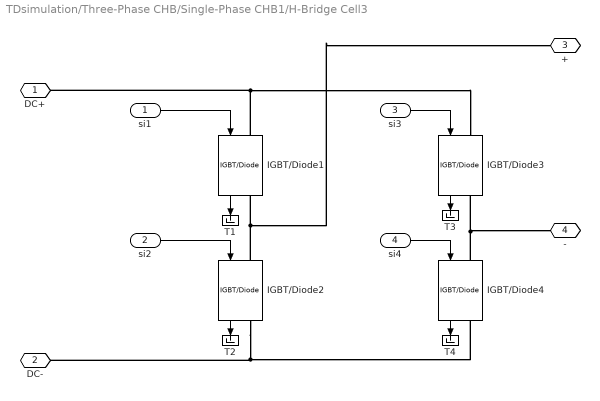
== system TDsimulation/Three-Phase CHB/Single-Phase CHB1/H-Bridge Cell3 ==
  si1 : Inport
  si2 : Inport  Port=2
  si3 : Inport  Port=3
  si4 : Inport  Port=4
  IGBT/Diode{1..4} (4 alike) : powerlib/Power Electronics/IGBT//Diode  Ron=1e-3  Rs=1e5  Cs=0.5  Measurements=on
  T{1..4} (4 alike) : Terminator
  DC+ : PMIOPort  Port=1  Side=Right
  DC- : PMIOPort  Port=2  Side=Right
  + : PMIOPort  Port=3  Side=Right
  - : PMIOPort  Port=4  Side=Right
  wires:
  si4/1 -> IGBT/Diode4/1
  si2/1 -> IGBT/Diode2/1
  si3/1 -> IGBT/Diode3/1
  si1/1 -> IGBT/Diode1/1
  IGBT/Diode1/1 -> T1/1
  IGBT/Diode2/1 -> T2/1
  IGBT/Diode4/1 -> T4/1
  IGBT/Diode3/1 -> T3/1
  connections:
  IGBT/Diode3/RConn1 -- IGBT/Diode4/LConn1 -- -/RConn1
  IGBT/Diode2/RConn1 -- IGBT/Diode4/RConn1 -- DC-/RConn1
  IGBT/Diode1/RConn1 -- IGBT/Diode2/LConn1 -- +/RConn1
  IGBT/Diode1/LConn1 -- IGBT/Diode3/LConn1 -- DC+/RConn1

== system TDsimulation/Three-Phase CHB/Single-Phase CHB1/H-Bridge Driver1 ==
  si1 : Inport
  si3 : Inport  Port=2
  Logical Operator2 : Logic  Operator=NOT  AllPortsSameDT=off  OutDataTypeStr=boolean
  Logical Operator3 : Logic  Operator=NOT  AllPortsSameDT=off  OutDataTypeStr=boolean
  1 : Outport
  2 : Outport  Port=2
  3 : Outport  Port=3
  4 : Outport  Port=4
  wires:
  si3/1 -> 3/1, Logical Operator3/1
  si1/1 -> 1/1, Logical Operator2/1
  Logical Operator3/1 -> 4/1
  Logical Operator2/1 -> 2/1

== system TDsimulation/Three-Phase CHB/Single-Phase CHB1/H-Bridge Driver2 ==
  si1 : Inport
  si3 : Inport  Port=2
  Logical Operator2 : Logic  Operator=NOT  AllPortsSameDT=off  OutDataTypeStr=boolean
  Logical Operator3 : Logic  Operator=NOT  AllPortsSameDT=off  OutDataTypeStr=boolean
  1 : Outport
  2 : Outport  Port=2
  3 : Outport  Port=3
  4 : Outport  Port=4
  wires:
  si3/1 -> 3/1, Logical Operator3/1
  si1/1 -> 1/1, Logical Operator2/1
  Logical Operator3/1 -> 4/1
  Logical Operator2/1 -> 2/1

== system TDsimulation/Three-Phase CHB/Single-Phase CHB1/H-Bridge Driver3 ==
  si1 : Inport
  si3 : Inport  Port=2
  Logical Operator2 : Logic  Operator=NOT  AllPortsSameDT=off  OutDataTypeStr=boolean
  Logical Operator3 : Logic  Operator=NOT  AllPortsSameDT=off  OutDataTypeStr=boolean
  1 : Outport
  2 : Outport  Port=2
  3 : Outport  Port=3
  4 : Outport  Port=4
  wires:
  si3/1 -> 3/1, Logical Operator3/1
  si1/1 -> 1/1, Logical Operator2/1
  Logical Operator3/1 -> 4/1
  Logical Operator2/1 -> 2/1

== system TDsimulation/Three-Phase CHB/Single-Phase CHB2/DC-Link1 ==
  Constant : Constant  Value=Ideal
  DC Capacitor : powerlib/Elements/Series RLC Branch  LConnTagsString=__new0  RConnTagsString=__new0  BranchType=C  Resistance=0.09  Inductance=0.002996  SetiL0=off  InitialCurrent=0  Capacitance=Cdc  Setx0=on  InitialVoltage=Vodc  Measurements=None
  DC Voltage Source : powerlib/Electrical Sources/DC Voltage Source  Amplitude=Vdc  Measurements=None
  Ideal Switch : powerlib/Power Electronics/Ideal Switch  Ron=0.001  Lon=0  IC=0  Rs=1e5  Cs=inf  Measurements=on
  Ideal Switch1 : powerlib/Power Electronics/Ideal Switch  Ron=0.001  Lon=0  IC=0  Rs=1e5  Cs=inf  Measurements=on
  Logical Operator2 : Logic  Operator=NOT  AllPortsSameDT=off  OutDataTypeStr=boolean
  Vcan3 : powerlib/Measurements/Voltage Measurement  PhasorSimulation=off  OutputType=Complex  PSBequivalent=0
  + : PMIOPort  Port=1  Side=Right
  - : PMIOPort  Port=2  Side=Right
  tag scope: Vccb1=global
  wires:
  Constant/1 -> Ideal Switch/1, Logical Operator2/1
  Logical Operator2/1 -> Ideal Switch1/1
  Vcan3/1 -> [Vccb1]
  connections:
  DC Capacitor/LConn1 -- Ideal Switch1/LConn1
  Ideal Switch1/RConn1 -- Ideal Switch/RConn1 -- Vcan3/LConn1 -- +/RConn1
  DC Voltage Source/RConn1 -- Ideal Switch/LConn1
  -/RConn1 -- Vcan3/LConn2 -- DC Capacitor/RConn1 -- DC Voltage Source/LConn1

== system TDsimulation/Three-Phase CHB/Single-Phase CHB2/DC-Link2 ==
  Constant : Constant  Value=Ideal
  DC Capacitor : powerlib/Elements/Series RLC Branch  LConnTagsString=__new0  RConnTagsString=__new0  BranchType=C  Resistance=0.09  Inductance=0.002996  SetiL0=off  InitialCurrent=0  Capacitance=Cdc  Setx0=on  InitialVoltage=Vodc  Measurements=None
  DC Voltage Source : powerlib/Electrical Sources/DC Voltage Source  Amplitude=Vdc  Measurements=None
  Ideal Switch : powerlib/Power Electronics/Ideal Switch  Ron=0.001  Lon=0  IC=0  Rs=1e5  Cs=inf  Measurements=on
  Ideal Switch1 : powerlib/Power Electronics/Ideal Switch  Ron=0.001  Lon=0  IC=0  Rs=1e5  Cs=inf  Measurements=on
  Logical Operator2 : Logic  Operator=NOT  AllPortsSameDT=off  OutDataTypeStr=boolean
  Vcan3 : powerlib/Measurements/Voltage Measurement  PhasorSimulation=off  OutputType=Complex  PSBequivalent=0
  + : PMIOPort  Port=1  Side=Right
  - : PMIOPort  Port=2  Side=Right
  tag scope: Vccb2=global
  wires:
  Constant/1 -> Ideal Switch/1, Logical Operator2/1
  Logical Operator2/1 -> Ideal Switch1/1
  Vcan3/1 -> [Vccb2]
  connections:
  DC Capacitor/LConn1 -- Ideal Switch1/LConn1
  Ideal Switch1/RConn1 -- Ideal Switch/RConn1 -- Vcan3/LConn1 -- +/RConn1
  DC Voltage Source/RConn1 -- Ideal Switch/LConn1
  -/RConn1 -- Vcan3/LConn2 -- DC Capacitor/RConn1 -- DC Voltage Source/LConn1

== system TDsimulation/Three-Phase CHB/Single-Phase CHB2/DC-Link3 ==
  Constant : Constant  Value=Ideal
  DC Capacitor : powerlib/Elements/Series RLC Branch  LConnTagsString=__new0  RConnTagsString=__new0  BranchType=C  Resistance=0.09  Inductance=0.002996  SetiL0=off  InitialCurrent=0  Capacitance=Cdc  Setx0=on  InitialVoltage=Vodc  Measurements=None
  DC Voltage Source : powerlib/Electrical Sources/DC Voltage Source  Amplitude=Vdc  Measurements=None
  Ideal Switch : powerlib/Power Electronics/Ideal Switch  Ron=0.001  Lon=0  IC=0  Rs=1e5  Cs=inf  Measurements=on
  Ideal Switch1 : powerlib/Power Electronics/Ideal Switch  Ron=0.001  Lon=0  IC=0  Rs=1e5  Cs=inf  Measurements=on
  Logical Operator2 : Logic  Operator=NOT  AllPortsSameDT=off  OutDataTypeStr=boolean
  Vcan3 : powerlib/Measurements/Voltage Measurement  PhasorSimulation=off  OutputType=Complex  PSBequivalent=0
  + : PMIOPort  Port=1  Side=Right
  - : PMIOPort  Port=2  Side=Right
  tag scope: Vccb3=global
  wires:
  Constant/1 -> Ideal Switch/1, Logical Operator2/1
  Logical Operator2/1 -> Ideal Switch1/1
  Vcan3/1 -> [Vccb3]
  connections:
  DC Capacitor/LConn1 -- Ideal Switch1/LConn1
  Ideal Switch1/RConn1 -- Ideal Switch/RConn1 -- Vcan3/LConn1 -- +/RConn1
  DC Voltage Source/RConn1 -- Ideal Switch/LConn1
  -/RConn1 -- Vcan3/LConn2 -- DC Capacitor/RConn1 -- DC Voltage Source/LConn1

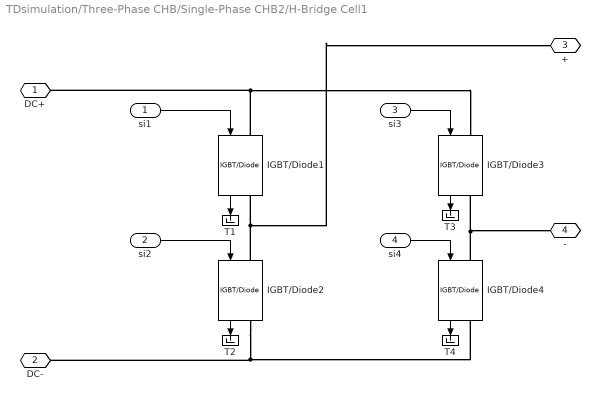
== system TDsimulation/Three-Phase CHB/Single-Phase CHB2/H-Bridge Cell1 ==
  si1 : Inport
  si2 : Inport  Port=2
  si3 : Inport  Port=3
  si4 : Inport  Port=4
  IGBT/Diode{1..4} (4 alike) : powerlib/Power Electronics/IGBT//Diode  Ron=1e-3  Rs=1e5  Cs=0.5  Measurements=on
  T{1..4} (4 alike) : Terminator
  DC+ : PMIOPort  Port=1  Side=Right
  DC- : PMIOPort  Port=2  Side=Right
  + : PMIOPort  Port=3  Side=Right
  - : PMIOPort  Port=4  Side=Right
  wires:
  si4/1 -> IGBT/Diode4/1
  si2/1 -> IGBT/Diode2/1
  si3/1 -> IGBT/Diode3/1
  si1/1 -> IGBT/Diode1/1
  IGBT/Diode1/1 -> T1/1
  IGBT/Diode2/1 -> T2/1
  IGBT/Diode4/1 -> T4/1
  IGBT/Diode3/1 -> T3/1
  connections:
  IGBT/Diode3/RConn1 -- IGBT/Diode4/LConn1 -- -/RConn1
  IGBT/Diode2/RConn1 -- IGBT/Diode4/RConn1 -- DC-/RConn1
  IGBT/Diode1/RConn1 -- IGBT/Diode2/LConn1 -- +/RConn1
  IGBT/Diode1/LConn1 -- IGBT/Diode3/LConn1 -- DC+/RConn1

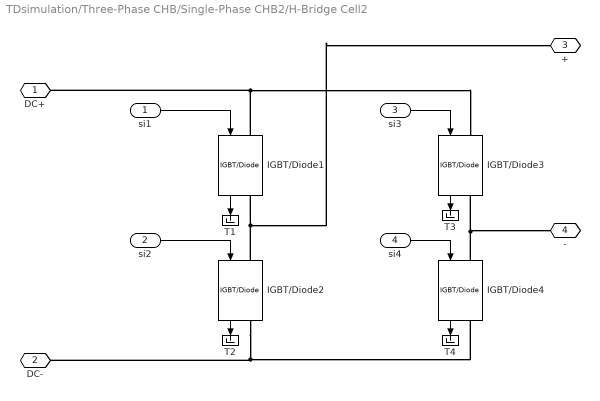
== system TDsimulation/Three-Phase CHB/Single-Phase CHB2/H-Bridge Cell2 ==
  si1 : Inport
  si2 : Inport  Port=2
  si3 : Inport  Port=3
  si4 : Inport  Port=4
  IGBT/Diode{1..4} (4 alike) : powerlib/Power Electronics/IGBT//Diode  Ron=1e-3  Rs=1e5  Cs=0.5  Measurements=on
  T{1..4} (4 alike) : Terminator
  DC+ : PMIOPort  Port=1  Side=Right
  DC- : PMIOPort  Port=2  Side=Right
  + : PMIOPort  Port=3  Side=Right
  - : PMIOPort  Port=4  Side=Right
  wires:
  si4/1 -> IGBT/Diode4/1
  si2/1 -> IGBT/Diode2/1
  si3/1 -> IGBT/Diode3/1
  si1/1 -> IGBT/Diode1/1
  IGBT/Diode1/1 -> T1/1
  IGBT/Diode2/1 -> T2/1
  IGBT/Diode4/1 -> T4/1
  IGBT/Diode3/1 -> T3/1
  connections:
  IGBT/Diode3/RConn1 -- IGBT/Diode4/LConn1 -- -/RConn1
  IGBT/Diode2/RConn1 -- IGBT/Diode4/RConn1 -- DC-/RConn1
  IGBT/Diode1/RConn1 -- IGBT/Diode2/LConn1 -- +/RConn1
  IGBT/Diode1/LConn1 -- IGBT/Diode3/LConn1 -- DC+/RConn1

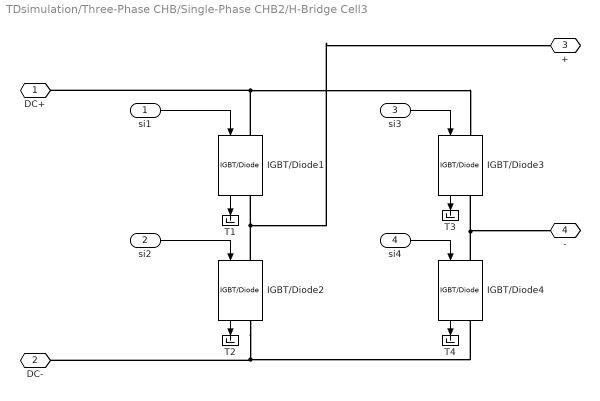
== system TDsimulation/Three-Phase CHB/Single-Phase CHB2/H-Bridge Cell3 ==
  si1 : Inport
  si2 : Inport  Port=2
  si3 : Inport  Port=3
  si4 : Inport  Port=4
  IGBT/Diode{1..4} (4 alike) : powerlib/Power Electronics/IGBT//Diode  Ron=1e-3  Rs=1e5  Cs=0.5  Measurements=on
  T{1..4} (4 alike) : Terminator
  DC+ : PMIOPort  Port=1  Side=Right
  DC- : PMIOPort  Port=2  Side=Right
  + : PMIOPort  Port=3  Side=Right
  - : PMIOPort  Port=4  Side=Right
  wires:
  si4/1 -> IGBT/Diode4/1
  si2/1 -> IGBT/Diode2/1
  si3/1 -> IGBT/Diode3/1
  si1/1 -> IGBT/Diode1/1
  IGBT/Diode1/1 -> T1/1
  IGBT/Diode2/1 -> T2/1
  IGBT/Diode4/1 -> T4/1
  IGBT/Diode3/1 -> T3/1
  connections:
  IGBT/Diode3/RConn1 -- IGBT/Diode4/LConn1 -- -/RConn1
  IGBT/Diode2/RConn1 -- IGBT/Diode4/RConn1 -- DC-/RConn1
  IGBT/Diode1/RConn1 -- IGBT/Diode2/LConn1 -- +/RConn1
  IGBT/Diode1/LConn1 -- IGBT/Diode3/LConn1 -- DC+/RConn1

== system TDsimulation/Three-Phase CHB/Single-Phase CHB2/H-Bridge Driver1 ==
  si1 : Inport
  si3 : Inport  Port=2
  Logical Operator2 : Logic  Operator=NOT  AllPortsSameDT=off  OutDataTypeStr=boolean
  Logical Operator3 : Logic  Operator=NOT  AllPortsSameDT=off  OutDataTypeStr=boolean
  1 : Outport
  2 : Outport  Port=2
  3 : Outport  Port=3
  4 : Outport  Port=4
  wires:
  si3/1 -> 3/1, Logical Operator3/1
  si1/1 -> 1/1, Logical Operator2/1
  Logical Operator3/1 -> 4/1
  Logical Operator2/1 -> 2/1

== system TDsimulation/Three-Phase CHB/Single-Phase CHB2/H-Bridge Driver2 ==
  si1 : Inport
  si3 : Inport  Port=2
  Logical Operator2 : Logic  Operator=NOT  AllPortsSameDT=off  OutDataTypeStr=boolean
  Logical Operator3 : Logic  Operator=NOT  AllPortsSameDT=off  OutDataTypeStr=boolean
  1 : Outport
  2 : Outport  Port=2
  3 : Outport  Port=3
  4 : Outport  Port=4
  wires:
  si3/1 -> 3/1, Logical Operator3/1
  si1/1 -> 1/1, Logical Operator2/1
  Logical Operator3/1 -> 4/1
  Logical Operator2/1 -> 2/1

== system TDsimulation/Three-Phase CHB/Single-Phase CHB2/H-Bridge Driver3 ==
  si1 : Inport
  si3 : Inport  Port=2
  Logical Operator2 : Logic  Operator=NOT  AllPortsSameDT=off  OutDataTypeStr=boolean
  Logical Operator3 : Logic  Operator=NOT  AllPortsSameDT=off  OutDataTypeStr=boolean
  1 : Outport
  2 : Outport  Port=2
  3 : Outport  Port=3
  4 : Outport  Port=4
  wires:
  si3/1 -> 3/1, Logical Operator3/1
  si1/1 -> 1/1, Logical Operator2/1
  Logical Operator3/1 -> 4/1
  Logical Operator2/1 -> 2/1

== system TDsimulation/Three-Phase CHB/Single-Phase CHB3/DC-Link1 ==
  Constant : Constant  Value=Ideal
  DC Capacitor : powerlib/Elements/Series RLC Branch  LConnTagsString=__new0  RConnTagsString=__new0  BranchType=C  Resistance=0.09  Inductance=0.002996  SetiL0=off  InitialCurrent=0  Capacitance=Cdc  Setx0=on  InitialVoltage=Vodc  Measurements=None
  DC Voltage Source : powerlib/Electrical Sources/DC Voltage Source  Amplitude=Vdc  Measurements=None
  Ideal Switch : powerlib/Power Electronics/Ideal Switch  Ron=0.001  Lon=0  IC=0  Rs=1e5  Cs=inf  Measurements=on
  Ideal Switch1 : powerlib/Power Electronics/Ideal Switch  Ron=0.001  Lon=0  IC=0  Rs=1e5  Cs=inf  Measurements=on
  Logical Operator2 : Logic  Operator=NOT  AllPortsSameDT=off  OutDataTypeStr=boolean
  Vcan3 : powerlib/Measurements/Voltage Measurement  PhasorSimulation=off  OutputType=Complex  PSBequivalent=0
  + : PMIOPort  Port=1  Side=Right
  - : PMIOPort  Port=2  Side=Right
  tag scope: Vccc1=global
  wires:
  Constant/1 -> Ideal Switch/1, Logical Operator2/1
  Logical Operator2/1 -> Ideal Switch1/1
  Vcan3/1 -> [Vccc1]
  connections:
  DC Capacitor/LConn1 -- Ideal Switch1/LConn1
  Ideal Switch1/RConn1 -- Ideal Switch/RConn1 -- Vcan3/LConn1 -- +/RConn1
  DC Voltage Source/RConn1 -- Ideal Switch/LConn1
  -/RConn1 -- Vcan3/LConn2 -- DC Capacitor/RConn1 -- DC Voltage Source/LConn1

== system TDsimulation/Three-Phase CHB/Single-Phase CHB3/DC-Link2 ==
  Constant : Constant  Value=Ideal
  DC Capacitor : powerlib/Elements/Series RLC Branch  LConnTagsString=__new0  RConnTagsString=__new0  BranchType=C  Resistance=0.09  Inductance=0.002996  SetiL0=off  InitialCurrent=0  Capacitance=Cdc  Setx0=on  InitialVoltage=Vodc  Measurements=None
  DC Voltage Source : powerlib/Electrical Sources/DC Voltage Source  Amplitude=Vdc  Measurements=None
  Ideal Switch : powerlib/Power Electronics/Ideal Switch  Ron=0.001  Lon=0  IC=0  Rs=1e5  Cs=inf  Measurements=on
  Ideal Switch1 : powerlib/Power Electronics/Ideal Switch  Ron=0.001  Lon=0  IC=0  Rs=1e5  Cs=inf  Measurements=on
  Logical Operator2 : Logic  Operator=NOT  AllPortsSameDT=off  OutDataTypeStr=boolean
  Vcan3 : powerlib/Measurements/Voltage Measurement  PhasorSimulation=off  OutputType=Complex  PSBequivalent=0
  + : PMIOPort  Port=1  Side=Right
  - : PMIOPort  Port=2  Side=Right
  tag scope: Vccc2=global
  wires:
  Constant/1 -> Ideal Switch/1, Logical Operator2/1
  Logical Operator2/1 -> Ideal Switch1/1
  Vcan3/1 -> [Vccc2]
  connections:
  DC Capacitor/LConn1 -- Ideal Switch1/LConn1
  Ideal Switch1/RConn1 -- Ideal Switch/RConn1 -- Vcan3/LConn1 -- +/RConn1
  DC Voltage Source/RConn1 -- Ideal Switch/LConn1
  -/RConn1 -- Vcan3/LConn2 -- DC Capacitor/RConn1 -- DC Voltage Source/LConn1

== system TDsimulation/Three-Phase CHB/Single-Phase CHB3/DC-Link3 ==
  Constant : Constant  Value=Ideal
  DC Capacitor : powerlib/Elements/Series RLC Branch  LConnTagsString=__new0  RConnTagsString=__new0  BranchType=C  Resistance=0.09  Inductance=0.002996  SetiL0=off  InitialCurrent=0  Capacitance=Cdc  Setx0=on  InitialVoltage=Vodc  Measurements=None
  DC Voltage Source : powerlib/Electrical Sources/DC Voltage Source  Amplitude=Vdc  Measurements=None
  Ideal Switch : powerlib/Power Electronics/Ideal Switch  Ron=0.001  Lon=0  IC=0  Rs=1e5  Cs=inf  Measurements=on
  Ideal Switch1 : powerlib/Power Electronics/Ideal Switch  Ron=0.001  Lon=0  IC=0  Rs=1e5  Cs=inf  Measurements=on
  Logical Operator2 : Logic  Operator=NOT  AllPortsSameDT=off  OutDataTypeStr=boolean
  Vcan3 : powerlib/Measurements/Voltage Measurement  PhasorSimulation=off  OutputType=Complex  PSBequivalent=0
  + : PMIOPort  Port=1  Side=Right
  - : PMIOPort  Port=2  Side=Right
  tag scope: Vccc3=global
  wires:
  Constant/1 -> Ideal Switch/1, Logical Operator2/1
  Logical Operator2/1 -> Ideal Switch1/1
  Vcan3/1 -> [Vccc3]
  connections:
  DC Capacitor/LConn1 -- Ideal Switch1/LConn1
  Ideal Switch1/RConn1 -- Ideal Switch/RConn1 -- Vcan3/LConn1 -- +/RConn1
  DC Voltage Source/RConn1 -- Ideal Switch/LConn1
  -/RConn1 -- Vcan3/LConn2 -- DC Capacitor/RConn1 -- DC Voltage Source/LConn1

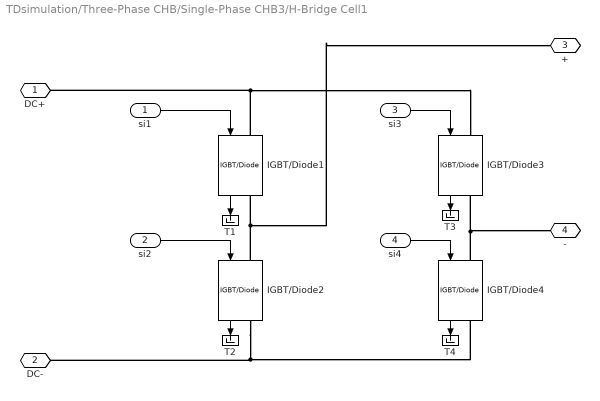
== system TDsimulation/Three-Phase CHB/Single-Phase CHB3/H-Bridge Cell1 ==
  si1 : Inport
  si2 : Inport  Port=2
  si3 : Inport  Port=3
  si4 : Inport  Port=4
  IGBT/Diode{1..4} (4 alike) : powerlib/Power Electronics/IGBT//Diode  Ron=1e-3  Rs=1e5  Cs=0.5  Measurements=on
  T{1..4} (4 alike) : Terminator
  DC+ : PMIOPort  Port=1  Side=Right
  DC- : PMIOPort  Port=2  Side=Right
  + : PMIOPort  Port=3  Side=Right
  - : PMIOPort  Port=4  Side=Right
  wires:
  si4/1 -> IGBT/Diode4/1
  si2/1 -> IGBT/Diode2/1
  si3/1 -> IGBT/Diode3/1
  si1/1 -> IGBT/Diode1/1
  IGBT/Diode1/1 -> T1/1
  IGBT/Diode2/1 -> T2/1
  IGBT/Diode4/1 -> T4/1
  IGBT/Diode3/1 -> T3/1
  connections:
  IGBT/Diode3/RConn1 -- IGBT/Diode4/LConn1 -- -/RConn1
  IGBT/Diode2/RConn1 -- IGBT/Diode4/RConn1 -- DC-/RConn1
  IGBT/Diode1/RConn1 -- IGBT/Diode2/LConn1 -- +/RConn1
  IGBT/Diode1/LConn1 -- IGBT/Diode3/LConn1 -- DC+/RConn1
